simulink model "sm_parts_ell_tubes"  (R2017b)
settings: Solver=VariableStepAuto  StartTime=0.0  StopTime=10.0  RelTol=1e-3  EnableMultiTasking=on
libraries: Multibody_Parts_Lib x3, sm_lib x2, nesl_utility x1
Description:
  | Copyright 2017-2018 The MathWorks, Inc.
settings Model: Creator=smiller  LastModifiedBy=smiller
settings DataIOCC: LimitDataPoints=on
settings OptimizationCC: LifeSpan=inf
settings DebuggingCC: AllowSymbolicDim=off  SFUnexpectedBacktrackingDiag=warning  SFNoUnconditionalDefaultTransitionDiag=warning  SFExecutionAtInitializationDiag=none
settings CodeAppCC: StateflowObjectComments=on
settings GRTTargetCC: TargetLangStandard=C89/C90 (ANSI)  GeneratePreprocessorConditionals=Disable all
settings ConfigComp: CovMetricSettings=dw  CovHtmlReporting=on  CovSaveCumulativeToWorkspaceVar=on  CovSaveSingleToWorkspaceVar=on  CovExternalEMLEnable=off  CovSFcnEnable=off
settings SimscapeCC: SimscapeNormalizeSystem=off  SimscapeLogType=all  SimscapeLogDataHistory=10000
settings ConfigurationSet: Description=SimMechanics 2G
settings ExplorerConfigSet: InternalSimMechanicsExplorerSettings="<ExplorerConfiguration><canonicalview>default</canonicalview><AnimationSetting><BasePlaybackSpeed>1.0</BasePlaybackSpeed><PlaybackSpeedFactor>1.0</PlaybackSpeedFactor></AnimationSetting><TilePanel><TileInfo><Tiles Columns=\"1\" Count=\"1\" Rows=\"1\"><Column Left=\"2\" Weight=\"1\"/><Column Left=\"429\"/><Row Top=\"2\" Weight=\"1\"/><Row Top=\"206\"/><Tile Height=\"1\" Width=\"1\" X=\"0\" Y=\"0\"/></Tiles></TileInfo><SceneInfo><SceneViewer><BGColor><R>1</R><G>1</G><B>1</B></BGColor><Camera><DoPerspective>off</DoPerspective><Position><X>0.69668420423490574</X><Y>0.13582902124554172</Y><Z>-0.27672864672645714</Z></Position><Center><X>-0.28238340476899482</X><Y>0.024908485658090562</Y><Z>-0.1060732870556324</Z></Center><Up><X>-0.1154830733610594</X><Y>0.99316372912511386</Y><Z>-0.017013727321820223</Z></Up><ViewLimDist>1</ViewLimDist><YLim>0.09653787264448889</YLim><XLim>0.20693759366869927</XLim></Camera></SceneViewer></SceneInfo></TilePanel><MechEditorPanel><Cameras/><GfxPanelCameraMap/><VideoCreator><PlaybackSpeedRatio>1.0</PlaybackSpeedRatio><FrameRate>30</FrameRate><VideoFormat>Motion JPEG AVI</VideoFormat><FrameSize>auto</FrameSize></VideoCreator></MechEditorPanel></ExplorerConfiguration>"

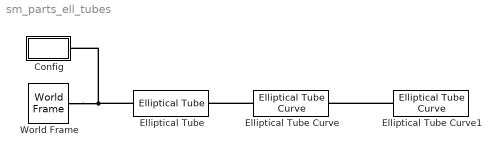
== system sm_parts_ell_tubes ==
  Config : Subsystem
  Elliptical Tube : Multibody_Parts_Lib/Extrusions/Elliptical Tube  rad_a=5e-2  rad_b=2e-2  deg_1=60  deg_2=315  ctr=0.5  ell_len=0.3  ell_rho=7000  ell_color=[0 0.4 0.6]  ell_opc=1
      settings: SourceProductName=Simscape Multibody Parts Library
  Elliptical Tube Curve : Multibody_Parts_Lib/Extrusions/Elliptical Tube Curve  rad_a=5e-2  rad_b=2e-2  deg_1=60  deg_2=315  ctr=0.5  arc_rad=0.15  arc_angle=115  popup_arcdir=Y  ell_rho=7000  ell_color=[0.8 0.8 0.8]  ell_opc=1
      settings: SourceProductName=Simscape Multibody Parts Library
  Elliptical Tube Curve1 : Multibody_Parts_Lib/Extrusions/Elliptical Tube Curve  rad_a=5e-2  rad_b=2e-2  deg_1=60  deg_2=315  ctr=0.5  arc_rad=0.03  arc_angle=180  popup_arcdir=Z  ell_rho=7000  ell_color=[0 0.4 0.6]  ell_opc=1
      settings: SourceProductName=Simscape Multibody Parts Library
  World Frame : sm_lib/Frames and Transforms/World Frame
  connections:
  World Frame/RConn1 -- Elliptical Tube/RConn1 -- Config/LConn1
  Elliptical Tube Curve1/RConn1 -- Elliptical Tube Curve/LConn1
  Elliptical Tube Curve/RConn1 -- Elliptical Tube/LConn1

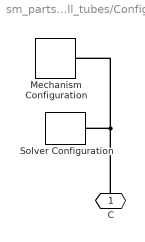
== system sm_parts_ell_tubes/Config ==
  Mechanism Configuration : sm_lib/Utilities/Mechanism Configuration  UniformGravity=Constant  GravityVector=[0 0 -9.80665]  GravityUnits=m/s^2  LinearizationDelta=0.001
  Solver Configuration : nesl_utility/Solver Configuration  PhysicalDomain=network_engine_domain  SubClassName=solver  LeftPortType=input  RightPortType=generic  Accelerate=off  Tones=[]  Harmonics=[]  SimulateNoise=off  Profile=off  UseLocalSampling=off  EnableSwitchedLinearOptims=on  FrequencyDomain=off  UseCCode=off  RelTol=0.001  AbsTol=1e-06  MinStep=1e-09  ToWorkspace=off  RevertToSquareIcSolve=off  NumHomotopyIterations=100  PhasorMode=off  PhasorModeNumHarmonics=1  DoDC=off  ResidualTolerance=1e-09  UseLocalSolver=off  LocalSolverChoice=NE_BACKWARD_EULER_ADVANCER  LocalSolverSampleTime=0.001  DoFixedCost=off  MaxNonlinIter=3  MaxModeIter=2  LinearAlgebra=Sparse  DelaysMemoryBudget=1024  AutomaticFiltering=on  FilteringTimeConstant=0.001
  C : PMIOPort  Port=1  Side=Left
  connections:
  Mechanism Configuration/RConn1 -- C/RConn1 -- Solver Configuration/RConn1
